simulink model "integrationModel"  (R2018b)
settings: Solver=FixedStepAuto  StartTime=0.0  StopTime=2  FixedStep=0.5  MaxStep=0.5  RelTol=1e-3
settings Model: Creator=Reichl  LastModifiedBy=Reichl
settings DataIOCC: FinalStateName=FinalStates  SaveFinalState=on  SaveFormat=Array  SaveState=on  StateSaveName=States
settings SFSimCC: SimUseLocalCustomCode=off
settings RTWCC: RTWUseLocalCustomCode=off
settings CodeAppCC: StateflowObjectComments=on

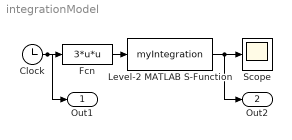
== system integrationModel ==
  Clock : Clock
  Fcn : Fcn  Expr=3*u*u
  Level-2 MATLAB S-Function : M-S-Function  FunctionName=myIntegration  Parameters=0.5
  Scope : Scope
  Out1 : Outport
  Out2 : Outport  Port=2
  wires:
  Level-2 MATLAB S-Function/1 -> Out2/1, Scope/1
  Clock/1 -> Out1/1, Fcn/1
  Fcn/1 -> Level-2 MATLAB S-Function/1
